simulink model "BMS_ClosedLoop"  (R2022b)
settings: configuration reference "BMS_Sw_CodeGenConfig" (kept outside this file)
values from neighbouring files (symbols this model uses):
  Ns_Module = 6.0    [Battery_16Packs_1RC.sldd]    (also in Battery_16Packs_3RC.sldd; Battery_1Pack_1RC.sldd; Battery_1Pack_3RC.sldd)
  NumModules = 16.0    [Battery_16Packs_1RC.sldd]    (also in Battery_16Packs_3RC.sldd; Battery_1Pack_1RC.sldd = 1.0; Battery_1Pack_3RC.sldd = 1.0)
CloseFcn:
  | cleanDictionaries
settings Model: DataDictionary=Battery_System_DD.sldd  EnableAccessToBaseWorkspace=off  PauseTimes=0  Creator=mluethy  LastModifiedBy=Loki
settings ConfigSetRef: SourceName=BMS_Sw_CodeGenConfig

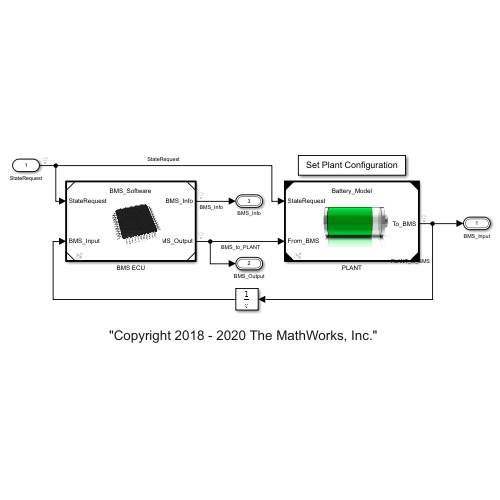
[thumbnail: Simulink's stored preview of the top-level diagram]
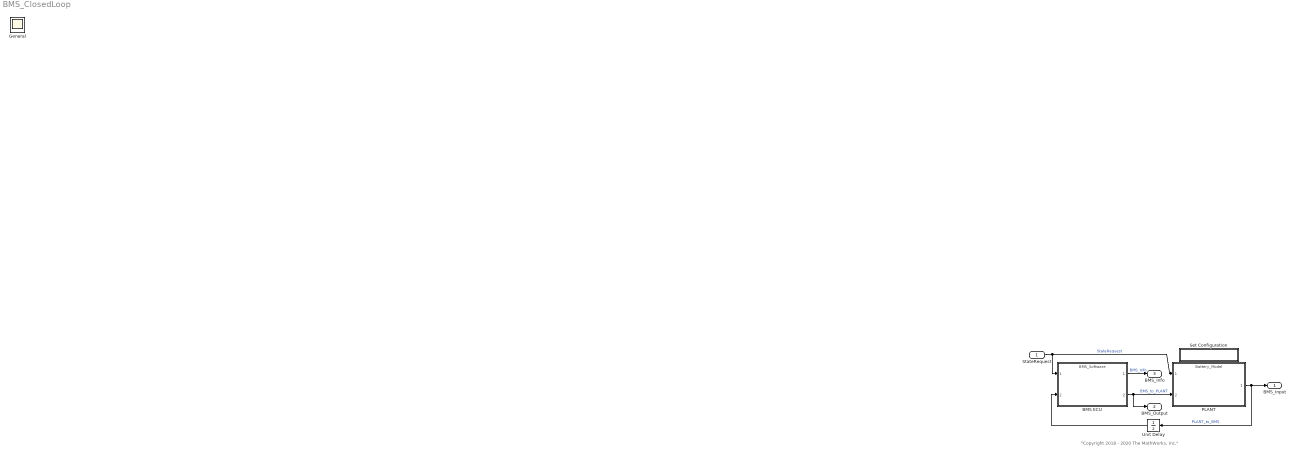
== system BMS_ClosedLoop ==
  note: "Copyright 2018 - 2020 The MathWorks, Inc."
  StateRequest : Inport  OutDataTypeStr=Enum: SRE
  BMS ECU : ModelReference  ModelNameDialog=BMS_Software  SimulationMode=Normal  ModelReferenceVersion=6.0
      mask Display: image('Microcontroller.jpg',[50,17,58,48])
  PLANT : ModelReference  ModelNameDialog=Battery_Model  ModelReferenceVersion=6.1
      mask Display: image('Plant_Battery.jpg',[40,15,80,48])
  Set Configuration : Subsystem
      mask Display: disp('Set Plant Configuration');
  Unit Delay : UnitDelay  InitialCondition=struct('Cell_Voltages',3.6*ones(1, Ns_Module*NumModules),'Pack_Voltage',3.6*Ns_Module*NumModules,'Pack_Current',0,'Vout_Chgr',0,'Vout_Invtr',0,'Cell_Temperatures',293.15*ones(1,Ns_Module*NumModules))  SampleTime=-1  HasFrameUpgradeWarning=on
  BMS_Input : Outport  OutDataTypeStr=Bus: BMS_Input  VectorParamsAs1DForOutWhenUnconnected=off
  BMS_Output : Outport  Port=2  OutDataTypeStr=Bus: BMS_Output  VectorParamsAs1DForOutWhenUnconnected=off
  BMS_Info : Outport  Port=3  OutDataTypeStr=Bus: BMS_Info  VectorParamsAs1DForOutWhenUnconnected=off  BusOutputAsStruct=on
  General : Scope
  wires:
  StateRequest/1 -> PLANT/1, BMS ECU/1  "StateRequest"
  PLANT/1 -> Unit Delay/1, BMS_Input/1  "PLANT_to_BMS"
  BMS ECU/1 -> BMS_Info/1  "BMS_Info"
  BMS ECU/2 -> PLANT/2, BMS_Output/1  "BMS_to_PLANT"
  Unit Delay/1 -> BMS ECU/2

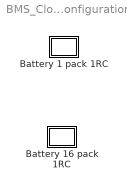
== system BMS_ClosedLoop/Set Configuration ==
  Battery 1 pack 1RC : Subsystem
      settings: OpenFcn=|
      | SharedDictionaryObj = Simulink.data.dictionary.open('Shared_DD.sldd');
      | try removeDataSource(SharedDictionaryObj,'Battery_1Pack_1RC.sldd')
      | end
      | try removeDataSource(SharedDictionaryObj,'Battery_16Packs_1RC.sldd')
      | end
      | addDataSource(SharedDictionaryObj,'Battery_1Pack_1RC.sldd')
  Battery 16 pack 1RC : Subsystem
      settings: OpenFcn=|
      | SharedDictionaryObj = Simulink.data.dictionary.open('Shared_DD.sldd');
      | try removeDataSource(SharedDictionaryObj,'Battery_1Pack_1RC.sldd')
      | end
      | try removeDataSource(SharedDictionaryObj,'Battery_16Packs_1RC.sldd')
      | end
      | addDataSource(SharedDictionaryObj,'Battery_16Packs_1RC.sldd')

== system BMS_ClosedLoop/Set Configuration/Battery 1 pack 1RC ==

== system BMS_ClosedLoop/Set Configuration/Battery 16 pack 1RC ==
